simulink model "data_cap"  (R2013b)
settings: Solver=ode45  StartTime=0.0  StopTime=270000  RelTol=1e-3
undefined symbols (not defined in the file or in its folder): A, A2, B, D, EVAL, i, P, THIS_DATE, W, X, Z
libraries: xbsIndex_r4 x219, uram_lib x2
(part 1 of 2)
settings Model: Creator=ehngjun  LastModifiedBy=Administrator
settings GRTTargetCC: CodeReplacementLibrary=C89/C90 (ANSI)

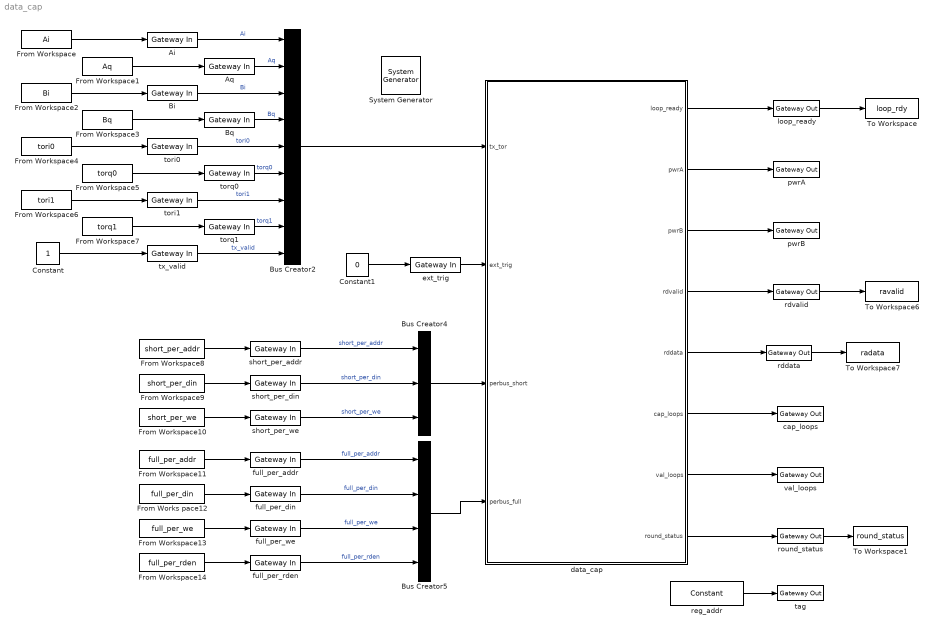
== system data_cap ==
  " System Generator" : xbsIndex_r4/ System Generator  Tag=genX  xilinxfamily=zynquplus  part=xczu15eg  speed=-1LV-i-EVAL  package=ffvb1156  synthesis_tool=Vivado  clock_wrapper=Clock Enables  directory=../../../netlist/datacap  proj_type=Vivado  Synth_file=Vivado Synthesis Defaults  Impl_file=Vivado Implementation Defaults  testbench=off  simulink_period=1  sysclk_period=3.2  dcm_input_clock_period=10  incr_netlist=off  trim_vbits=Everywhere in SubSystem  dbl_ovrd=According to Block Masks  core_generation=According to Block Masks  run_coregen=off  deprecated_control=off  eval_field=0  block_type=sysgen
  Ai : xbsIndex_r4/Gateway In  gui_display_data_type=Fixed-point  arith_type="Signed  (2's comp)"  n_bits=16  bin_pt=0  preci_type=Single  exp_width=8  frac_width=24  rows=1  columns=1  quantization="Round  (unbiased: +/- Inf)"  overflow=Saturate  period=1  UseAsADC=off  ADCChannel='1'  interface=None  automatic_assignment=on  address_offset=hex2dec('00')  intf_name=''  intf_description=''  default_value=0  timing_constraint=None  locs_specified=off  LOCs={}  io_standard={}  inherit_from_input=off  hdl_port=on  dbl_ovrd=off  block_type=gatewayin
  Aq : xbsIndex_r4/Gateway In  gui_display_data_type=Fixed-point  arith_type="Signed  (2's comp)"  n_bits=16  bin_pt=0  preci_type=Single  exp_width=8  frac_width=24  rows=1  columns=1  quantization="Round  (unbiased: +/- Inf)"  overflow=Saturate  period=1  UseAsADC=off  ADCChannel='1'  interface=None  automatic_assignment=on  address_offset=hex2dec('00')  intf_name=''  intf_description=''  default_value=0  timing_constraint=None  locs_specified=off  LOCs={}  io_standard={}  inherit_from_input=off  hdl_port=on  dbl_ovrd=off  block_type=gatewayin
  Bi : xbsIndex_r4/Gateway In  gui_display_data_type=Fixed-point  arith_type="Signed  (2's comp)"  n_bits=16  bin_pt=0  preci_type=Single  exp_width=8  frac_width=24  rows=1  columns=1  quantization="Round  (unbiased: +/- Inf)"  overflow=Saturate  period=1  UseAsADC=off  ADCChannel='1'  interface=None  automatic_assignment=on  address_offset=hex2dec('00')  intf_name=''  intf_description=''  default_value=0  timing_constraint=None  locs_specified=off  LOCs={}  io_standard={}  inherit_from_input=off  hdl_port=on  dbl_ovrd=off  block_type=gatewayin
  Bq : xbsIndex_r4/Gateway In  gui_display_data_type=Fixed-point  arith_type="Signed  (2's comp)"  n_bits=16  bin_pt=0  preci_type=Single  exp_width=8  frac_width=24  rows=1  columns=1  quantization="Round  (unbiased: +/- Inf)"  overflow=Saturate  period=1  UseAsADC=off  ADCChannel='1'  interface=None  automatic_assignment=on  address_offset=hex2dec('00')  intf_name=''  intf_description=''  default_value=0  timing_constraint=None  locs_specified=off  LOCs={}  io_standard={}  inherit_from_input=off  hdl_port=on  dbl_ovrd=off  block_type=gatewayin
  Bus Creator2 : BusCreator  Inputs=9
  Bus Creator4 : BusCreator  Inputs=3
  Bus Creator5 : BusCreator
  Constant : Constant
  Constant1 : Constant  Value=0
  From Works pace12 : FromWorkspace  VariableName=full_per_din  SampleTime=1  Interpolate=off  OutputAfterFinalValue=Setting to zero
  From Workspace : FromWorkspace  VariableName=Ai  SampleTime=1  Interpolate=off  OutputAfterFinalValue=Setting to zero
  From Workspace1 : FromWorkspace  VariableName=Aq  SampleTime=1  Interpolate=off  OutputAfterFinalValue=Setting to zero
  From Workspace10 : FromWorkspace  VariableName=short_per_we  SampleTime=1  Interpolate=off  OutputAfterFinalValue=Setting to zero
  From Workspace11 : FromWorkspace  VariableName=full_per_addr  SampleTime=1  Interpolate=off  OutputAfterFinalValue=Setting to zero
  From Workspace13 : FromWorkspace  VariableName=full_per_we  SampleTime=1  Interpolate=off  OutputAfterFinalValue=Setting to zero
  From Workspace14 : FromWorkspace  VariableName=full_per_rden  SampleTime=1  Interpolate=off  OutputAfterFinalValue=Setting to zero
  From Workspace2 : FromWorkspace  VariableName=Bi  SampleTime=1  Interpolate=off  OutputAfterFinalValue=Setting to zero
  From Workspace3 : FromWorkspace  VariableName=Bq  SampleTime=1  Interpolate=off  OutputAfterFinalValue=Setting to zero
  From Workspace4 : FromWorkspace  VariableName=tori0  SampleTime=1  Interpolate=off  OutputAfterFinalValue=Setting to zero
  From Workspace5 : FromWorkspace  VariableName=torq0  SampleTime=1  Interpolate=off  OutputAfterFinalValue=Setting to zero
  From Workspace6 : FromWorkspace  VariableName=tori1  SampleTime=1  Interpolate=off  OutputAfterFinalValue=Setting to zero
  From Workspace7 : FromWorkspace  VariableName=torq1  SampleTime=1  Interpolate=off  OutputAfterFinalValue=Setting to zero
  From Workspace8 : FromWorkspace  VariableName=short_per_addr  SampleTime=1  Interpolate=off  OutputAfterFinalValue=Setting to zero
  From Workspace9 : FromWorkspace  VariableName=short_per_din  SampleTime=1  Interpolate=off  OutputAfterFinalValue=Setting to zero
  To Workspace : ToWorkspace  VariableName=loop_rdy  SampleTime=-1
  To Workspace1 : ToWorkspace  VariableName=round_status  SampleTime=-1
  To Workspace6 : ToWorkspace  VariableName=ravalid  SampleTime=-1
  To Workspace7 : ToWorkspace  VariableName=radata  SampleTime=-1
  cap_loops : xbsIndex_r4/Gateway Out  inherit_from_input=off  hdl_port=on  rows=1  columns=1  UseAsDAC=off  DACChannel='1'  interface=None  automatic_assignment=on  address_offset=hex2dec('00')  intf_name=''  intf_description=''  timing_constraint=None  locs_specified=off  LOCs={}  io_standard={}  block_type=gatewayout
  data_cap : Subsystem
  ext_trig : xbsIndex_r4/Gateway In  gui_display_data_type=Boolean  arith_type=Boolean  n_bits=16  bin_pt=14  preci_type=Single  exp_width=8  frac_width=24  rows=1  columns=1  quantization="Round  (unbiased: +/- Inf)"  overflow=Saturate  period=1  UseAsADC=off  ADCChannel='1'  interface=None  automatic_assignment=on  address_offset=hex2dec('00')  intf_name=''  intf_description=''  default_value=0  timing_constraint=None  locs_specified=off  LOCs={}  io_standard={}  inherit_from_input=off  hdl_port=on  dbl_ovrd=off  block_type=gatewayin
  full_per_addr : xbsIndex_r4/Gateway In  gui_display_data_type=Fixed-point  arith_type=Unsigned  n_bits=20  bin_pt=0  preci_type=Single  exp_width=8  frac_width=24  rows=1  columns=1  quantization="Round  (unbiased: +/- Inf)"  overflow=Saturate  period=1  UseAsADC=off  ADCChannel='1'  interface=None  automatic_assignment=on  address_offset=hex2dec('00')  intf_name=''  intf_description=''  default_value=0  timing_constraint=None  locs_specified=off  LOCs={}  io_standard={}  inherit_from_input=off  hdl_port=on  dbl_ovrd=off  block_type=gatewayin
  full_per_din : xbsIndex_r4/Gateway In  gui_display_data_type=Fixed-point  arith_type=Unsigned  n_bits=32  bin_pt=0  preci_type=Single  exp_width=8  frac_width=24  rows=1  columns=1  quantization="Round  (unbiased: +/- Inf)"  overflow=Saturate  period=1  UseAsADC=off  ADCChannel='1'  interface=None  automatic_assignment=on  address_offset=hex2dec('00')  intf_name=''  intf_description=''  default_value=0  timing_constraint=None  locs_specified=off  LOCs={}  io_standard={}  inherit_from_input=off  hdl_port=on  dbl_ovrd=off  block_type=gatewayin
  full_per_rden : xbsIndex_r4/Gateway In  gui_display_data_type=Boolean  arith_type=Boolean  n_bits=16  bin_pt=0  preci_type=Single  exp_width=8  frac_width=24  rows=1  columns=1  quantization="Round  (unbiased: +/- Inf)"  overflow=Saturate  period=1  UseAsADC=off  ADCChannel='1'  interface=None  automatic_assignment=on  address_offset=hex2dec('00')  intf_name=''  intf_description=''  default_value=0  timing_constraint=None  locs_specified=off  LOCs={}  io_standard={}  inherit_from_input=off  hdl_port=on  dbl_ovrd=off  block_type=gatewayin
  full_per_we : xbsIndex_r4/Gateway In  gui_display_data_type=Boolean  arith_type=Boolean  n_bits=16  bin_pt=0  preci_type=Single  exp_width=8  frac_width=24  rows=1  columns=1  quantization="Round  (unbiased: +/- Inf)"  overflow=Saturate  period=1  UseAsADC=off  ADCChannel='1'  interface=None  automatic_assignment=on  address_offset=hex2dec('00')  intf_name=''  intf_description=''  default_value=0  timing_constraint=None  locs_specified=off  LOCs={}  io_standard={}  inherit_from_input=off  hdl_port=on  dbl_ovrd=off  block_type=gatewayin
  loop_ready : xbsIndex_r4/Gateway Out  inherit_from_input=off  hdl_port=on  rows=1  columns=1  UseAsDAC=off  DACChannel='1'  interface=None  automatic_assignment=on  address_offset=hex2dec('00')  intf_name=''  intf_description=''  timing_constraint=None  locs_specified=off  LOCs={}  io_standard={}  block_type=gatewayout
  pwrA : xbsIndex_r4/Gateway Out  inherit_from_input=off  hdl_port=on  rows=1  columns=1  UseAsDAC=off  DACChannel='1'  interface=None  automatic_assignment=on  address_offset=hex2dec('00')  intf_name=''  intf_description=''  timing_constraint=None  locs_specified=off  LOCs={}  io_standard={}  block_type=gatewayout
  pwrB : xbsIndex_r4/Gateway Out  inherit_from_input=off  hdl_port=on  rows=1  columns=1  UseAsDAC=off  DACChannel='1'  interface=None  automatic_assignment=on  address_offset=hex2dec('00')  intf_name=''  intf_description=''  timing_constraint=None  locs_specified=off  LOCs={}  io_standard={}  block_type=gatewayout
  rddata : xbsIndex_r4/Gateway Out  inherit_from_input=off  hdl_port=on  rows=1  columns=1  UseAsDAC=off  DACChannel='1'  interface=None  automatic_assignment=on  address_offset=hex2dec('00')  intf_name=''  intf_description=''  timing_constraint=None  locs_specified=off  LOCs={}  io_standard={}  block_type=gatewayout
  rdvalid : xbsIndex_r4/Gateway Out  inherit_from_input=off  hdl_port=on  rows=1  columns=1  UseAsDAC=off  DACChannel='1'  interface=None  automatic_assignment=on  address_offset=hex2dec('00')  intf_name=''  intf_description=''  timing_constraint=None  locs_specified=off  LOCs={}  io_standard={}  block_type=gatewayout
  reg_addr : xbsIndex_r4/Constant  const=THIS_DATE  gui_display_data_type=Fixed-point  arith_type=Unsigned  n_bits=32  bin_pt=0  preci_type=Single  exp_width=8  frac_width=24  explicit_period=off  period=1  equ=P=C  opselect=C  inp2=PCIN>>17  opr=+  inp1=P  carry=CIN  dbl_ovrd=off  block_type=constant
  round_status : xbsIndex_r4/Gateway Out  inherit_from_input=off  hdl_port=on  rows=1  columns=1  UseAsDAC=off  DACChannel='1'  interface=None  automatic_assignment=on  address_offset=hex2dec('00')  intf_name=''  intf_description=''  timing_constraint=None  locs_specified=off  LOCs={}  io_standard={}  block_type=gatewayout
  short_per_addr : xbsIndex_r4/Gateway In  gui_display_data_type=Fixed-point  arith_type=Unsigned  n_bits=12  bin_pt=0  preci_type=Single  exp_width=8  frac_width=24  rows=1  columns=1  quantization="Round  (unbiased: +/- Inf)"  overflow=Saturate  period=1  UseAsADC=off  ADCChannel='1'  interface=None  automatic_assignment=on  address_offset=hex2dec('00')  intf_name=''  intf_description=''  default_value=0  timing_constraint=None  locs_specified=off  LOCs={}  io_standard={}  inherit_from_input=off  hdl_port=on  dbl_ovrd=off  block_type=gatewayin
  short_per_din : xbsIndex_r4/Gateway In  gui_display_data_type=Fixed-point  arith_type=Unsigned  n_bits=32  bin_pt=0  preci_type=Single  exp_width=8  frac_width=24  rows=1  columns=1  quantization="Round  (unbiased: +/- Inf)"  overflow=Saturate  period=1  UseAsADC=off  ADCChannel='1'  interface=None  automatic_assignment=on  address_offset=hex2dec('00')  intf_name=''  intf_description=''  default_value=0  timing_constraint=None  locs_specified=off  LOCs={}  io_standard={}  inherit_from_input=off  hdl_port=on  dbl_ovrd=off  block_type=gatewayin
  short_per_we : xbsIndex_r4/Gateway In  gui_display_data_type=Boolean  arith_type=Boolean  n_bits=16  bin_pt=0  preci_type=Single  exp_width=8  frac_width=24  rows=1  columns=1  quantization="Round  (unbiased: +/- Inf)"  overflow=Saturate  period=1  UseAsADC=off  ADCChannel='1'  interface=None  automatic_assignment=on  address_offset=hex2dec('00')  intf_name=''  intf_description=''  default_value=0  timing_constraint=None  locs_specified=off  LOCs={}  io_standard={}  inherit_from_input=off  hdl_port=on  dbl_ovrd=off  block_type=gatewayin
  tag : xbsIndex_r4/Gateway Out  inherit_from_input=off  hdl_port=on  rows=1  columns=1  UseAsDAC=off  DACChannel='1'  interface=None  automatic_assignment=on  address_offset=hex2dec('00')  intf_name=''  intf_description=''  timing_constraint=None  locs_specified=off  LOCs={}  io_standard={}  block_type=gatewayout
  tori0 : xbsIndex_r4/Gateway In  gui_display_data_type=Fixed-point  arith_type="Signed  (2's comp)"  n_bits=16  bin_pt=0  preci_type=Single  exp_width=8  frac_width=24  rows=1  columns=1  quantization="Round  (unbiased: +/- Inf)"  overflow=Saturate  period=1  UseAsADC=off  ADCChannel='1'  interface=None  automatic_assignment=on  address_offset=hex2dec('00')  intf_name=''  intf_description=''  default_value=0  timing_constraint=None  locs_specified=off  LOCs={}  io_standard={}  inherit_from_input=off  hdl_port=on  dbl_ovrd=off  block_type=gatewayin
  tori1 : xbsIndex_r4/Gateway In  gui_display_data_type=Fixed-point  arith_type="Signed  (2's comp)"  n_bits=16  bin_pt=0  preci_type=Single  exp_width=8  frac_width=24  rows=1  columns=1  quantization="Round  (unbiased: +/- Inf)"  overflow=Saturate  period=1  UseAsADC=off  ADCChannel='1'  interface=None  automatic_assignment=on  address_offset=hex2dec('00')  intf_name=''  intf_description=''  default_value=0  timing_constraint=None  locs_specified=off  LOCs={}  io_standard={}  inherit_from_input=off  hdl_port=on  dbl_ovrd=off  block_type=gatewayin
  torq0 : xbsIndex_r4/Gateway In  gui_display_data_type=Fixed-point  arith_type="Signed  (2's comp)"  n_bits=16  bin_pt=0  preci_type=Single  exp_width=8  frac_width=24  rows=1  columns=1  quantization="Round  (unbiased: +/- Inf)"  overflow=Saturate  period=1  UseAsADC=off  ADCChannel='1'  interface=None  automatic_assignment=on  address_offset=hex2dec('00')  intf_name=''  intf_description=''  default_value=0  timing_constraint=None  locs_specified=off  LOCs={}  io_standard={}  inherit_from_input=off  hdl_port=on  dbl_ovrd=off  block_type=gatewayin
  torq1 : xbsIndex_r4/Gateway In  gui_display_data_type=Fixed-point  arith_type="Signed  (2's comp)"  n_bits=16  bin_pt=0  preci_type=Single  exp_width=8  frac_width=24  rows=1  columns=1  quantization="Round  (unbiased: +/- Inf)"  overflow=Saturate  period=1  UseAsADC=off  ADCChannel='1'  interface=None  automatic_assignment=on  address_offset=hex2dec('00')  intf_name=''  intf_description=''  default_value=0  timing_constraint=None  locs_specified=off  LOCs={}  io_standard={}  inherit_from_input=off  hdl_port=on  dbl_ovrd=off  block_type=gatewayin
  tx_valid : xbsIndex_r4/Gateway In  gui_display_data_type=Boolean  arith_type=Boolean  n_bits=16  bin_pt=14  preci_type=Single  exp_width=8  frac_width=24  rows=1  columns=1  quantization="Round  (unbiased: +/- Inf)"  overflow=Saturate  period=1  UseAsADC=off  ADCChannel='1'  interface=None  automatic_assignment=on  address_offset=hex2dec('00')  intf_name=''  intf_description=''  default_value=0  timing_constraint=None  locs_specified=off  LOCs={}  io_standard={}  inherit_from_input=off  hdl_port=on  dbl_ovrd=off  block_type=gatewayin
  val_loops : xbsIndex_r4/Gateway Out  inherit_from_input=off  hdl_port=on  rows=1  columns=1  UseAsDAC=off  DACChannel='1'  interface=None  automatic_assignment=on  address_offset=hex2dec('00')  intf_name=''  intf_description=''  timing_constraint=None  locs_specified=off  LOCs={}  io_standard={}  block_type=gatewayout
  wires:
  Ai/1 -> Bus Creator2/1  "Ai"
  Bi/1 -> Bus Creator2/3  "Bi"
  tori0/1 -> Bus Creator2/5  "tori0"
  tori1/1 -> Bus Creator2/7  "tori1"
  Aq/1 -> Bus Creator2/2  "Aq"
  Bq/1 -> Bus Creator2/4  "Bq"
  torq0/1 -> Bus Creator2/6  "torq0"
  torq1/1 -> Bus Creator2/8  "torq1"
  tx_valid/1 -> Bus Creator2/9  "tx_valid"
  Bus Creator2/1 -> data_cap/1(tx_tor)
  ext_trig/1 -> data_cap/2(ext_trig)
  data_cap/8(round_status) -> round_status/1
  data_cap/6(cap_loops) -> cap_loops/1
  data_cap/7(val_loops) -> val_loops/1
  data_cap/2(pwrA) -> pwrA/1
  From Workspace/1 -> Ai/1
  From Workspace1/1 -> Aq/1
  From Workspace2/1 -> Bi/1
  From Workspace3/1 -> Bq/1
  From Workspace4/1 -> tori0/1
  From Workspace5/1 -> torq0/1
  From Workspace6/1 -> tori1/1
  From Workspace7/1 -> torq1/1
  Constant1/1 -> ext_trig/1
  loop_ready/1 -> To Workspace/1
  round_status/1 -> To Workspace1/1
  Constant/1 -> tx_valid/1
  data_cap/3(pwrB) -> pwrB/1
  short_per_addr/1 -> Bus Creator4/1  "short_per_addr"
  short_per_din/1 -> Bus Creator4/2  "short_per_din"
  short_per_we/1 -> Bus Creator4/3  "short_per_we"
  Bus Creator4/1 -> data_cap/3(perbus_short)
  full_per_addr/1 -> Bus Creator5/1  "full_per_addr"
  full_per_din/1 -> Bus Creator5/2  "full_per_din"
  full_per_we/1 -> Bus Creator5/3  "full_per_we"
  Bus Creator5/1 -> data_cap/4(perbus_full)
  data_cap/4(rdvalid) -> rdvalid/1
  rdvalid/1 -> To Workspace6/1
  From Workspace8/1 -> short_per_addr/1
  From Workspace9/1 -> short_per_din/1
  From Workspace10/1 -> short_per_we/1
  From Workspace11/1 -> full_per_addr/1
  From Works pace12/1 -> full_per_din/1
  From Workspace13/1 -> full_per_we/1
  data_cap/1(loop_ready) -> loop_ready/1
  data_cap/5(rddata) -> rddata/1
  rddata/1 -> To Workspace7/1
  From Workspace14/1 -> full_per_rden/1
  full_per_rden/1 -> Bus Creator5/4  "full_per_rden"
  reg_addr/1 -> tag/1

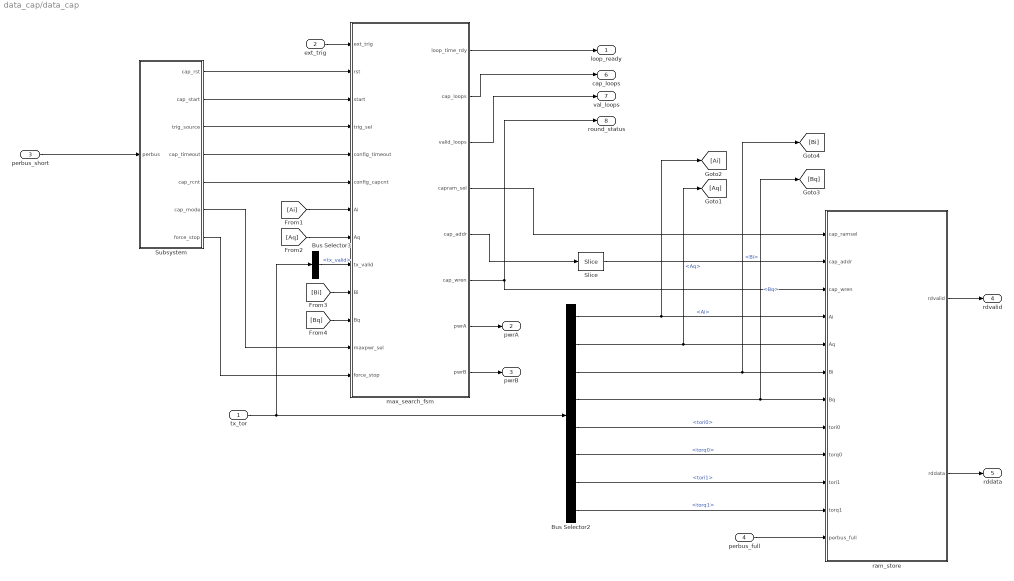
== system data_cap/data_cap ==
  tx_tor : Inport
  ext_trig : Inport  Port=2
  perbus_short : Inport  Port=3
  perbus_full : Inport  Port=4
  Bus Selector2 : BusSelector  OutputSignals=Ai,Aq,Bi,Bq,tori0,torq0,tori1,torq1
  Bus Selector3 : BusSelector  OutputSignals=tx_valid
  Slice : xbsIndex_r4/Slice  nbits=15  boolean_output=off  mode=Lower Bit Location + Width  bit1=0  base1=MSB of Input  bit0=0  base0=LSB of Input  dbl_ovrd=off  block_type=slice
  Subsystem : Subsystem
  max_search_fsm : Subsystem
  ram_store : Subsystem
  loop_ready : Outport
  pwrA : Outport  Port=2
  pwrB : Outport  Port=3
  rdvalid : Outport  Port=4
  rddata : Outport  Port=5
  cap_loops : Outport  Port=6
  val_loops : Outport  Port=7
  round_status : Outport  Port=8
  wires:
  Bus Selector3/1 -> max_search_fsm/9(tx_valid)  "<tx_valid>"
  [Aq] -> max_search_fsm/8(Aq)
  [Ai] -> max_search_fsm/7(Ai)
  Bus Selector2/5 -> ram_store/8(tori0)  "<tori0>"
  Bus Selector2/4 -> [Bq], ram_store/7(Bq)  "<Bq>"
  Bus Selector2/3 -> [Bi], ram_store/6(Bi)  "<Bi>"
  Bus Selector2/2 -> [Aq], ram_store/5(Aq)  "<Aq>"
  Bus Selector2/1 -> [Ai], ram_store/4(Ai)  "<Ai>"
  tx_tor/1 -> Bus Selector2/1, Bus Selector3/1
  Slice/1 -> ram_store/2(cap_addr)
  max_search_fsm/6(cap_wren) -> round_status/1, ram_store/3(cap_wren)
  max_search_fsm/5(cap_addr) -> Slice/1
  max_search_fsm/4(capram_sel) -> ram_store/1(cap_ramsel)
  max_search_fsm/3(valid_loops) -> val_loops/1
  max_search_fsm/2(cap_loops) -> cap_loops/1
  max_search_fsm/1(loop_time_rdy) -> loop_ready/1
  Subsystem/5(cap_rcnt) -> max_search_fsm/6(config_capcnt)
  Subsystem/4(cap_timeout) -> max_search_fsm/5(config_timeout)
  ext_trig/1 -> max_search_fsm/1(ext_trig)
  Subsystem/3(trig_source) -> max_search_fsm/4(trig_sel)
  Subsystem/2(cap_start) -> max_search_fsm/3(start)
  Bus Selector2/6 -> ram_store/9(torq0)  "<torq0>"
  Bus Selector2/7 -> ram_store/10(tori1)  "<tori1>"
  Bus Selector2/8 -> ram_store/11(torq1)  "<torq1>"
  [Bi] -> max_search_fsm/10(Bi)
  [Bq] -> max_search_fsm/11(Bq)
  Subsystem/6(cap_mode) -> max_search_fsm/12(maxpwr_sel)
  Subsystem/7(force_stop) -> max_search_fsm/13(force_stop)
  max_search_fsm/7(pwrA) -> pwrA/1
  max_search_fsm/8(pwrB) -> pwrB/1
  perbus_short/1 -> Subsystem/1(perbus)
  perbus_full/1 -> ram_store/12(perbus_full)
  ram_store/1(rdvalid) -> rdvalid/1
  ram_store/2(rddata) -> rddata/1
  Subsystem/1(cap_rst) -> max_search_fsm/2(rst)

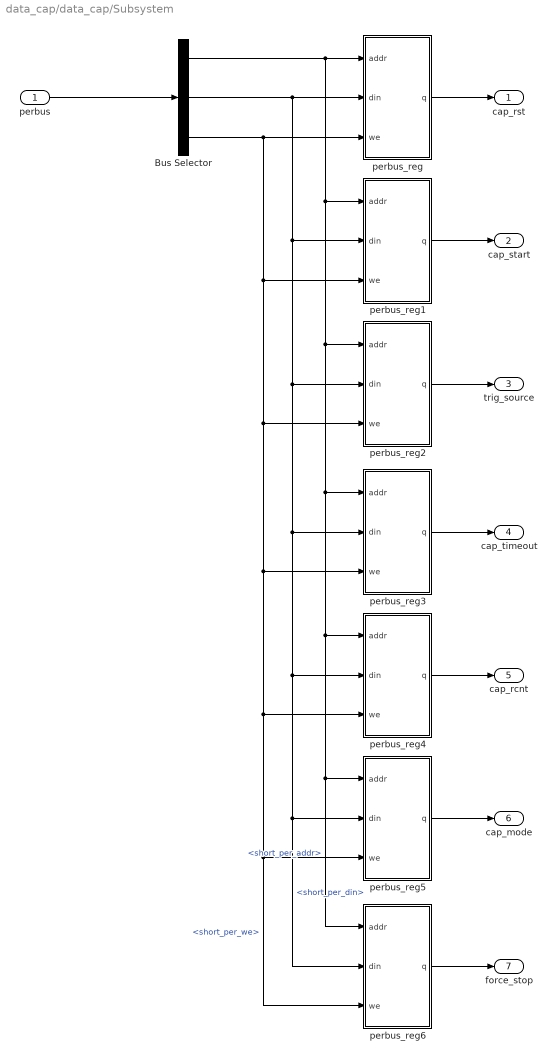
== system data_cap/data_cap/Subsystem ==
  perbus : Inport
  Bus Selector : BusSelector  OutputSignals=short_per_addr,short_per_din,short_per_we
  perbus_reg : Subsystem  mask{reg_addr=hex2dec('150')}
      mask prompts: reg_addr "cap_rst"
  perbus_reg1 : Subsystem  mask{reg_addr=hex2dec('150')}
      mask prompts: reg_addr "cap_start"
  perbus_reg2 : Subsystem  mask{reg_addr=hex2dec('150')}
      mask prompts: reg_addr "trig_source"
  perbus_reg3 : Subsystem  mask{reg_addr=hex2dec('152')}
      mask prompts: reg_addr "cap_timeout"
  perbus_reg4 : Subsystem  mask{reg_addr=hex2dec('151')}
      mask prompts: reg_addr "cap_rcnt"
  perbus_reg5 : Subsystem  mask{reg_addr=hex2dec('150')}
      mask prompts: reg_addr "cap_mode"
  perbus_reg6 : Subsystem  mask{reg_addr=hex2dec('150')}
      mask prompts: reg_addr "force_stop"
  cap_rst : Outport
  cap_start : Outport  Port=2
  trig_source : Outport  Port=3
  cap_timeout : Outport  Port=4
  cap_rcnt : Outport  Port=5
  cap_mode : Outport  Port=6
  force_stop : Outport  Port=7
  wires:
  perbus_reg/1(q) -> cap_rst/1
  Bus Selector/3 -> perbus_reg3/3(we), perbus_reg6/3(we), perbus_reg5/3(we), perbus_reg4/3(we), perbus_reg2/3(we), perbus_reg1/3(we), perbus_reg/3(we)  "<short_per_we>"
  Bus Selector/2 -> perbus_reg6/2(din), perbus_reg5/2(din), perbus_reg4/2(din), perbus_reg3/2(din), perbus_reg2/2(din), perbus_reg1/2(din), perbus_reg/2(din)  "<short_per_din>"
  Bus Selector/1 -> perbus_reg6/1(addr), perbus_reg5/1(addr), perbus_reg4/1(addr), perbus_reg3/1(addr), perbus_reg2/1(addr), perbus_reg1/1(addr), perbus_reg/1(addr)  "<short_per_addr>"
  perbus/1 -> Bus Selector/1
  perbus_reg6/1(q) -> force_stop/1
  perbus_reg5/1(q) -> cap_mode/1
  perbus_reg4/1(q) -> cap_rcnt/1
  perbus_reg1/1(q) -> cap_start/1
  perbus_reg2/1(q) -> trig_source/1
  perbus_reg3/1(q) -> cap_timeout/1

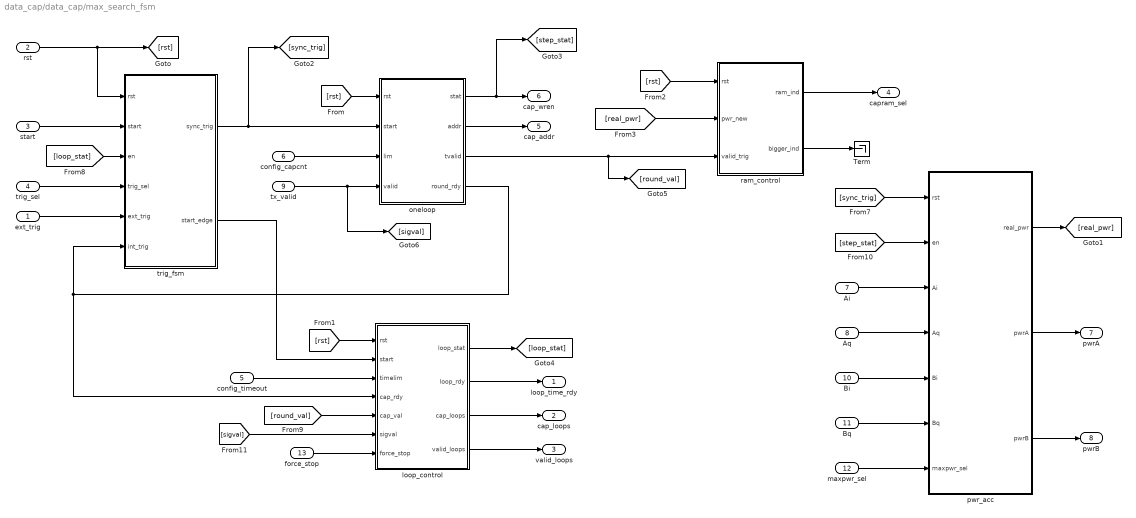
== system data_cap/data_cap/max_search_fsm ==
  ext_trig : Inport
  rst : Inport  Port=2
  start : Inport  Port=3
  trig_sel : Inport  Port=4
  config_timeout : Inport  Port=5
  config_capcnt : Inport  Port=6
  Ai : Inport  Port=7
  Aq : Inport  Port=8
  tx_valid : Inport  Port=9
  Bi : Inport  Port=10
  Bq : Inport  Port=11
  maxpwr_sel : Inport  Port=12
  force_stop : Inport  Port=13
  Term : Terminator
  loop_control : Subsystem
  oneloop : Subsystem
  pwr_acc : Subsystem
  ram_control : Subsystem
  trig_fsm : Subsystem
  loop_time_rdy : Outport
  cap_loops : Outport  Port=2
  valid_loops : Outport  Port=3
  capram_sel : Outport  Port=4
  cap_addr : Outport  Port=5
  cap_wren : Outport  Port=6
  pwrA : Outport  Port=7
  pwrB : Outport  Port=8
  wires:
  [step_stat] -> pwr_acc/2(en)
  tx_valid/1 -> [sigval], oneloop/4(valid)
  loop_control/4(valid_loops) -> valid_loops/1
  loop_control/3(cap_loops) -> cap_loops/1
  loop_control/2(loop_rdy) -> loop_time_rdy/1
  oneloop/1(stat) -> [step_stat], cap_wren/1
  oneloop/2(addr) -> cap_addr/1
  ram_control/2(bigger_ind) -> Term/1
  [round_val] -> loop_control/5(cap_val)
  [loop_stat] -> trig_fsm/3(en)
  loop_control/1(loop_stat) -> [loop_stat]
  Aq/1 -> pwr_acc/4(Aq)
  Ai/1 -> pwr_acc/3(Ai)
  [real_pwr] -> ram_control/2(pwr_new)
  pwr_acc/1(real_pwr) -> [real_pwr]
  oneloop/3(tvalid) -> ram_control/3(valid_trig), [round_val]
  [rst] -> ram_control/1(rst)
  config_timeout/1 -> loop_control/3(timelim)
  [rst] -> loop_control/1(rst)
  [rst] -> oneloop/1(rst)
  oneloop/4(round_rdy) -> loop_control/4(cap_rdy), trig_fsm/6(int_trig)
  config_capcnt/1 -> oneloop/3(lim)
  trig_fsm/1(sync_trig) -> oneloop/2(start), [sync_trig]
  ext_trig/1 -> trig_fsm/5(ext_trig)
  trig_sel/1 -> trig_fsm/4(trig_sel)
  start/1 -> trig_fsm/2(start)
  rst/1 -> trig_fsm/1(rst), [rst]
  [sigval] -> loop_control/6(sigval)
  Bi/1 -> pwr_acc/5(Bi)
  Bq/1 -> pwr_acc/6(Bq)
  maxpwr_sel/1 -> pwr_acc/7(maxpwr_sel)
  force_stop/1 -> loop_control/7(force_stop)
  pwr_acc/2(pwrA) -> pwrA/1
  pwr_acc/3(pwrB) -> pwrB/1
  trig_fsm/2(start_edge) -> loop_control/2(start)
  ram_control/1(ram_ind) -> capram_sel/1
  [sync_trig] -> pwr_acc/1(rst)

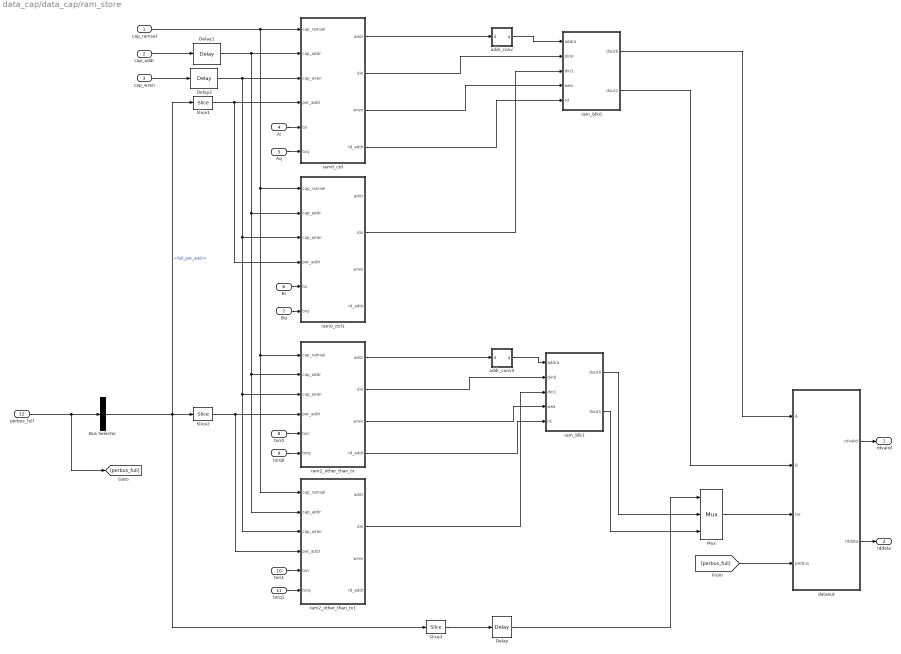
== system data_cap/data_cap/ram_store ==
  cap_ramsel : Inport
  cap_addr : Inport  Port=2
  cap_wren : Inport  Port=3
  Ai : Inport  Port=4
  Aq : Inport  Port=5
  Bi : Inport  Port=6
  Bq : Inport  Port=7
  tori0 : Inport  Port=8
  torq0 : Inport  Port=9
  tori1 : Inport  Port=10
  torq1 : Inport  Port=11
  perbus_full : Inport  Port=12
  Bus Selector : BusSelector  OutputSignals=full_per_addr
  Delay : xbsIndex_r4/Delay  rst=off  infoeditControl=Selection of Reset will increase slice count due to use of real FFs and instead of SRLs  en=off  latency=12  reg_retiming=off  dbl_ovrd=off  block_type=delay
  Delay1 : xbsIndex_r4/Delay  rst=off  infoeditControl=Selection of Reset will increase slice count due to use of real FFs and instead of SRLs  en=off  latency=1  reg_retiming=off  dbl_ovrd=off  block_type=delay
  Delay2 : xbsIndex_r4/Delay  rst=off  infoeditControl=Selection of Reset will increase slice count due to use of real FFs and instead of SRLs  en=off  latency=1  reg_retiming=off  dbl_ovrd=off  block_type=delay
  Mux : xbsIndex_r4/Mux  inputs=2  en=off  latency=0  precision=Full  arith_type=Unsigned  n_bits=16  bin_pt=14  quantization=Truncate  overflow=Wrap  dbl_ovrd=off  block_type=mux
  Slice1 : xbsIndex_r4/Slice  nbits=14  boolean_output=off  mode=Lower Bit Location + Width  bit1=0  base1=MSB of Input  bit0=0  base0=LSB of Input  dbl_ovrd=off  block_type=slice
  Slice2 : xbsIndex_r4/Slice  nbits=14  boolean_output=off  mode=Lower Bit Location + Width  bit1=0  base1=MSB of Input  bit0=1  base0=LSB of Input  dbl_ovrd=off  block_type=slice
  Slice3 : xbsIndex_r4/Slice  nbits=1  boolean_output=off  mode=Lower Bit Location + Width  bit1=0  base1=MSB of Input  bit0=0  base0=LSB of Input  dbl_ovrd=off  block_type=slice
  addr_conv : Subsystem  mask{cap_addr_width=14}
  addr_conv5 : Subsystem  mask{cap_addr_width=14}
  dataout : Subsystem
  ram0_ctrl : Subsystem
  ram0_ctrl1 : Subsystem
  ram2_other_than_tx : Subsystem
  ram2_other_than_tx1 : Subsystem
  ram_blk0 : Subsystem
  ram_blk1 : Subsystem
  rdvalid : Outport
  rddata : Outport  Port=2
  wires:
  Slice1/1 -> ram0_ctrl1/4(per_addr), ram0_ctrl/4(per_addr)
  ram2_other_than_tx/3(wren) -> ram_blk1/4(wea)
  ram2_other_than_tx/1(addr) -> addr_conv5/1(d)
  tori0/1 -> ram2_other_than_tx/5(tori)
  cap_ramsel/1 -> ram2_other_than_tx1/1(cap_ramsel), ram2_other_than_tx/1(cap_ramsel), ram0_ctrl1/1(cap_ramsel), ram0_ctrl/1(cap_ramsel)
  ram0_ctrl/3(wren) -> ram_blk0/4(wea)
  ram0_ctrl/2(din) -> ram_blk0/2(din0)
  ram0_ctrl/1(addr) -> addr_conv/1(d)
  Bq/1 -> ram0_ctrl1/6(txq)
  Bi/1 -> ram0_ctrl1/5(txi)
  Aq/1 -> ram0_ctrl/6(txq)
  cap_wren/1 -> Delay2/1
  addr_conv/1(q) -> ram_blk0/1(addra)
  ram2_other_than_tx/2(din) -> ram_blk1/2(din0)
  addr_conv5/1(q) -> ram_blk1/1(addra)
  ram2_other_than_tx/4(rd_addr) -> ram_blk1/5(rd)
  torq0/1 -> ram2_other_than_tx/6(torq)
  tori1/1 -> ram2_other_than_tx1/5(tori)
  torq1/1 -> ram2_other_than_tx1/6(torq)
  ram2_other_than_tx1/2(din) -> ram_blk1/3(din1)
  ram0_ctrl/4(rd_addr) -> ram_blk0/5(rd)
  Slice2/1 -> ram2_other_than_tx1/4(per_addr), ram2_other_than_tx/4(per_addr)
  dataout/2(rddata) -> rddata/1
  [perbus_full] -> dataout/4(perbus)
  ram_blk0/2(dout1) -> dataout/2(B)
  dataout/1(rdvalid) -> rdvalid/1
  perbus_full/1 -> [perbus_full], Bus Selector/1
  Bus Selector/1 -> Slice1/1, Slice3/1, Slice2/1  "<full_per_addr>"
  Slice3/1 -> Delay/1
  ram_blk1/1(dout0) -> Mux/2
  Mux/1 -> dataout/3(tor)
  Delay/1 -> Mux/1
  ram_blk0/1(dout0) -> dataout/1(A)
  Ai/1 -> ram0_ctrl/5(txi)
  Delay1/1 -> ram0_ctrl1/2(cap_addr), ram2_other_than_tx1/2(cap_addr), ram2_other_than_tx/2(cap_addr), ram0_ctrl/2(cap_addr)
  Delay2/1 -> ram0_ctrl1/3(cap_wren), ram2_other_than_tx1/3(cap_wren), ram2_other_than_tx/3(cap_wren), ram0_ctrl/3(cap_wren)
  ram_blk1/2(dout1) -> Mux/3
  cap_addr/1 -> Delay1/1
  ram0_ctrl1/2(din) -> ram_blk0/3(din1)

== system data_cap/data_cap/Subsystem/perbus_reg ==
  addr : Inport
  din : Inport  Port=2
  we : Inport  Port=3
  Logical : xbsIndex_r4/Logical  logical_function=AND  inputs=2  en=off  latency=0  precision=Full  arith_type=Unsigned  n_bits=16  bin_pt=0  align_bp=on  dbl_ovrd=off  block_type=logical
  Register : xbsIndex_r4/Register  init=0  rst=off  en=on  dbl_ovrd=off  block_type=register
  Relational : xbsIndex_r4/Relational  mode=a=b  op_type=Bool  en=off  latency=0  dbl_ovrd=off  block_type=relational
  bit[1] : xbsIndex_r4/Slice  nbits=1  boolean_output=on  mode=Lower Bit Location + Width  bit1=0  base1=MSB of Input  bit0=1  base0=LSB of Input  dbl_ovrd=off  block_type=slice
  reg_addr : xbsIndex_r4/Constant  const=reg_addr  gui_display_data_type=Fixed-point  arith_type=Unsigned  n_bits=12  bin_pt=0  preci_type=Single  exp_width=8  frac_width=24  explicit_period=off  period=1  equ=P=C  opselect=C  inp2=PCIN>>17  opr=+  inp1=P  carry=CIN  dbl_ovrd=off  block_type=constant
  q : Outport
  wires:
  reg_addr/1 -> Relational/2
  addr/1 -> Relational/1
  Relational/1 -> Logical/2
  we/1 -> Logical/1
  Logical/1 -> Register/2
  din/1 -> bit[1]/1
  Register/1 -> q/1
  bit[1]/1 -> Register/1

== system data_cap/data_cap/Subsystem/perbus_reg1 ==
  addr : Inport
  din : Inport  Port=2
  we : Inport  Port=3
  Logical : xbsIndex_r4/Logical  logical_function=AND  inputs=2  en=off  latency=0  precision=Full  arith_type=Unsigned  n_bits=16  bin_pt=0  align_bp=on  dbl_ovrd=off  block_type=logical
  Register : xbsIndex_r4/Register  init=0  rst=off  en=on  dbl_ovrd=off  block_type=register
  Relational : xbsIndex_r4/Relational  mode=a=b  op_type=Bool  en=off  latency=0  dbl_ovrd=off  block_type=relational
  bit[2] : xbsIndex_r4/Slice  nbits=1  boolean_output=on  mode=Lower Bit Location + Width  bit1=0  base1=MSB of Input  bit0=2  base0=LSB of Input  dbl_ovrd=off  block_type=slice
  reg_addr : xbsIndex_r4/Constant  const=reg_addr  gui_display_data_type=Fixed-point  arith_type=Unsigned  n_bits=12  bin_pt=0  preci_type=Single  exp_width=8  frac_width=24  explicit_period=off  period=1  equ=P=C  opselect=C  inp2=PCIN>>17  opr=+  inp1=P  carry=CIN  dbl_ovrd=off  block_type=constant
  q : Outport
  wires:
  Register/1 -> q/1
  din/1 -> bit[2]/1
  Logical/1 -> Register/2
  we/1 -> Logical/1
  Relational/1 -> Logical/2
  addr/1 -> Relational/1
  reg_addr/1 -> Relational/2
  bit[2]/1 -> Register/1

== system data_cap/data_cap/Subsystem/perbus_reg2 ==
  addr : Inport
  din : Inport  Port=2
  we : Inport  Port=3
  Logical : xbsIndex_r4/Logical  logical_function=AND  inputs=2  en=off  latency=0  precision=Full  arith_type=Unsigned  n_bits=16  bin_pt=0  align_bp=on  dbl_ovrd=off  block_type=logical
  Register : xbsIndex_r4/Register  init=0  rst=off  en=on  dbl_ovrd=off  block_type=register
  Relational : xbsIndex_r4/Relational  mode=a=b  op_type=Bool  en=off  latency=0  dbl_ovrd=off  block_type=relational
  bit[0] : xbsIndex_r4/Slice  nbits=1  boolean_output=on  mode=Lower Bit Location + Width  bit1=0  base1=MSB of Input  bit0=0  base0=LSB of Input  dbl_ovrd=off  block_type=slice
  reg_addr : xbsIndex_r4/Constant  const=reg_addr  gui_display_data_type=Fixed-point  arith_type=Unsigned  n_bits=12  bin_pt=0  preci_type=Single  exp_width=8  frac_width=24  explicit_period=off  period=1  equ=P=C  opselect=C  inp2=PCIN>>17  opr=+  inp1=P  carry=CIN  dbl_ovrd=off  block_type=constant
  q : Outport
  wires:
  reg_addr/1 -> Relational/2
  addr/1 -> Relational/1
  Relational/1 -> Logical/2
  we/1 -> Logical/1
  Logical/1 -> Register/2
  din/1 -> bit[0]/1
  Register/1 -> q/1
  bit[0]/1 -> Register/1

== system data_cap/data_cap/Subsystem/perbus_reg3 ==
  addr : Inport
  din : Inport  Port=2
  we : Inport  Port=3
  Logical : xbsIndex_r4/Logical  logical_function=AND  inputs=2  en=off  latency=0  precision=Full  arith_type=Unsigned  n_bits=16  bin_pt=0  align_bp=on  dbl_ovrd=off  block_type=logical
  Register : xbsIndex_r4/Register  init=0  rst=off  en=on  dbl_ovrd=off  block_type=register
  Relational : xbsIndex_r4/Relational  mode=a=b  op_type=Bool  en=off  latency=0  dbl_ovrd=off  block_type=relational
  reg_addr : xbsIndex_r4/Constant  const=reg_addr  gui_display_data_type=Fixed-point  arith_type=Unsigned  n_bits=12  bin_pt=0  preci_type=Single  exp_width=8  frac_width=24  explicit_period=off  period=1  equ=P=C  opselect=C  inp2=PCIN>>17  opr=+  inp1=P  carry=CIN  dbl_ovrd=off  block_type=constant
  q : Outport
  wires:
  Register/1 -> q/1
  din/1 -> Register/1
  Logical/1 -> Register/2
  we/1 -> Logical/1
  Relational/1 -> Logical/2
  addr/1 -> Relational/1
  reg_addr/1 -> Relational/2

== system data_cap/data_cap/Subsystem/perbus_reg4 ==
  addr : Inport
  din : Inport  Port=2
  we : Inport  Port=3
  Logical : xbsIndex_r4/Logical  logical_function=AND  inputs=2  en=off  latency=0  precision=Full  arith_type=Unsigned  n_bits=16  bin_pt=0  align_bp=on  dbl_ovrd=off  block_type=logical
  Register : xbsIndex_r4/Register  init=0  rst=off  en=on  dbl_ovrd=off  block_type=register
  Relational : xbsIndex_r4/Relational  mode=a=b  op_type=Bool  en=off  latency=0  dbl_ovrd=off  block_type=relational
  reg_addr : xbsIndex_r4/Constant  const=reg_addr  gui_display_data_type=Fixed-point  arith_type=Unsigned  n_bits=12  bin_pt=0  preci_type=Single  exp_width=8  frac_width=24  explicit_period=off  period=1  equ=P=C  opselect=C  inp2=PCIN>>17  opr=+  inp1=P  carry=CIN  dbl_ovrd=off  block_type=constant
  q : Outport
  wires:
  reg_addr/1 -> Relational/2
  addr/1 -> Relational/1
  Relational/1 -> Logical/2
  we/1 -> Logical/1
  Logical/1 -> Register/2
  din/1 -> Register/1
  Register/1 -> q/1

== system data_cap/data_cap/Subsystem/perbus_reg5 ==
  addr : Inport
  din : Inport  Port=2
  we : Inport  Port=3
  Logical : xbsIndex_r4/Logical  logical_function=AND  inputs=2  en=off  latency=0  precision=Full  arith_type=Unsigned  n_bits=16  bin_pt=0  align_bp=on  dbl_ovrd=off  block_type=logical
  Register : xbsIndex_r4/Register  init=0  rst=off  en=on  dbl_ovrd=off  block_type=register
  Relational : xbsIndex_r4/Relational  mode=a=b  op_type=Bool  en=off  latency=0  dbl_ovrd=off  block_type=relational
  bit[5-4] : xbsIndex_r4/Slice  nbits=2  boolean_output=off  mode=Lower Bit Location + Width  bit1=0  base1=MSB of Input  bit0=4  base0=LSB of Input  dbl_ovrd=off  block_type=slice
  reg_addr : xbsIndex_r4/Constant  const=reg_addr  gui_display_data_type=Fixed-point  arith_type=Unsigned  n_bits=12  bin_pt=0  preci_type=Single  exp_width=8  frac_width=24  explicit_period=off  period=1  equ=P=C  opselect=C  inp2=PCIN>>17  opr=+  inp1=P  carry=CIN  dbl_ovrd=off  block_type=constant
  q : Outport
  wires:
  Register/1 -> q/1
  din/1 -> bit[5-4]/1
  Logical/1 -> Register/2
  we/1 -> Logical/1
  Relational/1 -> Logical/2
  addr/1 -> Relational/1
  reg_addr/1 -> Relational/2
  bit[5-4]/1 -> Register/1

== system data_cap/data_cap/Subsystem/perbus_reg6 ==
  addr : Inport
  din : Inport  Port=2
  we : Inport  Port=3
  Logical : xbsIndex_r4/Logical  logical_function=AND  inputs=2  en=off  latency=0  precision=Full  arith_type=Unsigned  n_bits=16  bin_pt=0  align_bp=on  dbl_ovrd=off  block_type=logical
  Register : xbsIndex_r4/Register  init=0  rst=off  en=on  dbl_ovrd=off  block_type=register
  Relational : xbsIndex_r4/Relational  mode=a=b  op_type=Bool  en=off  latency=0  dbl_ovrd=off  block_type=relational
  bit[2] : xbsIndex_r4/Slice  nbits=1  boolean_output=on  mode=Lower Bit Location + Width  bit1=0  base1=MSB of Input  bit0=3  base0=LSB of Input  dbl_ovrd=off  block_type=slice
  reg_addr : xbsIndex_r4/Constant  const=reg_addr  gui_display_data_type=Fixed-point  arith_type=Unsigned  n_bits=12  bin_pt=0  preci_type=Single  exp_width=8  frac_width=24  explicit_period=off  period=1  equ=P=C  opselect=C  inp2=PCIN>>17  opr=+  inp1=P  carry=CIN  dbl_ovrd=off  block_type=constant
  q : Outport
  wires:
  reg_addr/1 -> Relational/2
  addr/1 -> Relational/1
  Relational/1 -> Logical/2
  we/1 -> Logical/1
  Logical/1 -> Register/2
  din/1 -> bit[2]/1
  Register/1 -> q/1
  bit[2]/1 -> Register/1

== system data_cap/data_cap/max_search_fsm/loop_control ==
  rst : Inport
  start : Inport  Port=2
  timelim : Inport  Port=3
  cap_rdy : Inport  Port=4
  cap_val : Inport  Port=5
  sigval : Inport  Port=6
  force_stop : Inport  Port=7
  cap_loop : xbsIndex_r4/Counter  cnt_type=Free Running  cnt_to=Inf  operation=Up  start_count=0  cnt_by_val=1  arith_type=Unsigned  n_bits=16  bin_pt=0  load_pin=off  rst=on  en=on  explicit_period=on  period=1  use_behavioral_HDL=off  implementation=Fabric  dbl_ovrd=off  block_type=counter
  time_counters : Subsystem
  valid_loop : xbsIndex_r4/Counter  cnt_type=Free Running  cnt_to=Inf  operation=Up  start_count=0  cnt_by_val=1  arith_type=Unsigned  n_bits=16  bin_pt=0  load_pin=off  rst=on  en=on  explicit_period=on  period=1  use_behavioral_HDL=off  implementation=Fabric  dbl_ovrd=off  block_type=counter
  loop_stat : Outport
  loop_rdy : Outport  Port=2
  cap_loops : Outport  Port=3
  valid_loops : Outport  Port=4
  wires:
  time_counters/2(rdy) -> loop_rdy/1
  time_counters/1(stat) -> loop_stat/1
  valid_loop/1 -> valid_loops/1
  cap_loop/1 -> cap_loops/1
  timelim/1 -> time_counters/3(timelim)
  start/1 -> time_counters/2(start)
  cap_val/1 -> valid_loop/2
  cap_rdy/1 -> cap_loop/2
  rst/1 -> valid_loop/1, cap_loop/1, time_counters/1(rst)
  sigval/1 -> time_counters/4(sigval)
  force_stop/1 -> time_counters/5(force_stop)

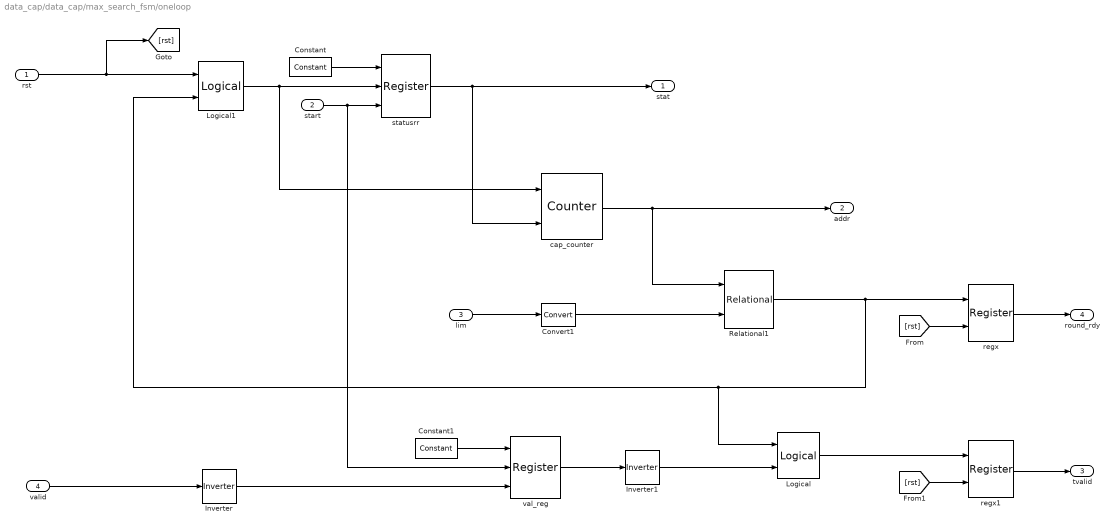
== system data_cap/data_cap/max_search_fsm/oneloop ==
  rst : Inport
  start : Inport  Port=2
  lim : Inport  Port=3
  valid : Inport  Port=4
  Constant : xbsIndex_r4/Constant  const=1  gui_display_data_type=Boolean  arith_type=Boolean  n_bits=1  bin_pt=0  preci_type=Single  exp_width=8  frac_width=24  explicit_period=off  period=1  equ=P=C  opselect=C  inp2=PCIN>>17  opr=+  inp1=P  carry=CIN  dbl_ovrd=off  block_type=constant
  Constant1 : xbsIndex_r4/Constant  const=1  gui_display_data_type=Boolean  arith_type=Boolean  n_bits=1  bin_pt=0  preci_type=Single  exp_width=8  frac_width=24  explicit_period=off  period=1  equ=P=C  opselect=C  inp2=PCIN>>17  opr=+  inp1=P  carry=CIN  dbl_ovrd=off  block_type=constant
  Convert1 : xbsIndex_r4/Convert  gui_display_data_type=Fixed-point  arith_type=Unsigned  n_bits=18  bin_pt=0  float_type=Single  exp_bits=8  fraction_bits=24  quantization=Truncate  overflow=Wrap  en=off  latency=0  pipeline=off  dbl_ovrd=off  block_type=convert
  Inverter : xbsIndex_r4/Inverter  en=off  latency=0  dbl_ovrd=off  block_type=inv
  Inverter1 : xbsIndex_r4/Inverter  en=off  latency=0  dbl_ovrd=off  block_type=inv
  Logical : xbsIndex_r4/Logical  logical_function=AND  inputs=2  en=off  latency=0  precision=Full  arith_type=Unsigned  n_bits=16  bin_pt=0  align_bp=on  dbl_ovrd=off  block_type=logical
  Logical1 : xbsIndex_r4/Logical  logical_function=OR  inputs=2  en=off  latency=0  precision=Full  arith_type=Unsigned  n_bits=16  bin_pt=0  align_bp=on  dbl_ovrd=off  block_type=logical
  Relational1 : xbsIndex_r4/Relational  mode=a=b  op_type=Bool  en=off  latency=0  dbl_ovrd=off  block_type=relational
  cap_counter : xbsIndex_r4/Counter  cnt_type=Free Running  cnt_to=Inf  operation=Up  start_count=0  cnt_by_val=1  arith_type=Unsigned  n_bits=18  bin_pt=0  load_pin=off  rst=on  en=on  explicit_period=on  period=1  use_behavioral_HDL=off  implementation=Fabric  dbl_ovrd=off  block_type=counter
  regx : xbsIndex_r4/Register  init=0  rst=on  en=off  dbl_ovrd=off  block_type=register
  regx1 : xbsIndex_r4/Register  init=0  rst=on  en=off  dbl_ovrd=off  block_type=register
  statusrr : xbsIndex_r4/Register  init=0  rst=on  en=on  dbl_ovrd=off  block_type=register
  val_reg : xbsIndex_r4/Register  init=0  rst=on  en=on  dbl_ovrd=off  block_type=register
  stat : Outport
  addr : Outport  Port=2
  tvalid : Outport  Port=3
  round_rdy : Outport  Port=4
  wires:
  [rst] -> regx1/2
  Logical/1 -> regx1/1
  [rst] -> regx/2
  regx/1 -> round_rdy/1
  val_reg/1 -> Inverter1/1
  Inverter/1 -> val_reg/3
  Constant1/1 -> val_reg/1
  start/1 -> val_reg/2, statusrr/3
  Constant/1 -> statusrr/1
  Logical1/1 -> statusrr/2, cap_counter/1
  rst/1 -> Logical1/1, [rst]
  Convert1/1 -> Relational1/2
  lim/1 -> Convert1/1
  Relational1/1 -> Logical1/2, Logical/1, regx/1
  valid/1 -> Inverter/1
  cap_counter/1 -> Relational1/1, addr/1
  statusrr/1 -> cap_counter/2, stat/1
  regx1/1 -> tvalid/1
  Inverter1/1 -> Logical/2

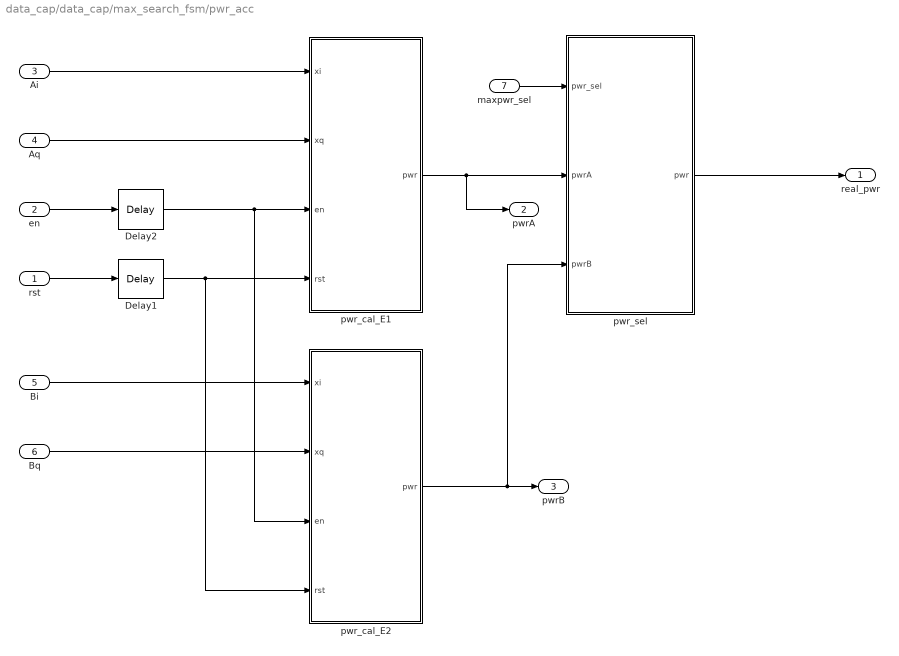
== system data_cap/data_cap/max_search_fsm/pwr_acc ==
  rst : Inport
  en : Inport  Port=2
  Ai : Inport  Port=3
  Aq : Inport  Port=4
  Bi : Inport  Port=5
  Bq : Inport  Port=6
  maxpwr_sel : Inport  Port=7
  Delay1 : xbsIndex_r4/Delay  rst=off  infoeditControl=Selection of Reset will increase slice count due to use of real FFs and instead of SRLs  en=off  latency=1  reg_retiming=off  dbl_ovrd=off  block_type=delay
  Delay2 : xbsIndex_r4/Delay  rst=off  infoeditControl=Selection of Reset will increase slice count due to use of real FFs and instead of SRLs  en=off  latency=1  reg_retiming=off  dbl_ovrd=off  block_type=delay
  pwr_cal_E1 : Subsystem
  pwr_cal_E2 : Subsystem
  pwr_sel : Subsystem
  real_pwr : Outport
  pwrA : Outport  Port=2
  pwrB : Outport  Port=3
  wires:
  en/1 -> Delay2/1
  rst/1 -> Delay1/1
  pwr_sel/1(pwr) -> real_pwr/1
  Ai/1 -> pwr_cal_E1/1(xi)
  Delay2/1 -> pwr_cal_E2/3(en), pwr_cal_E1/3(en)
  Delay1/1 -> pwr_cal_E2/4(rst), pwr_cal_E1/4(rst)
  Aq/1 -> pwr_cal_E1/2(xq)
  Bi/1 -> pwr_cal_E2/1(xi)
  Bq/1 -> pwr_cal_E2/2(xq)
  pwr_cal_E1/1(pwr) -> pwrA/1, pwr_sel/2(pwrA)
  pwr_cal_E2/1(pwr) -> pwrB/1, pwr_sel/3(pwrB)
  maxpwr_sel/1 -> pwr_sel/1(pwr_sel)

== system data_cap/data_cap/max_search_fsm/ram_control ==
  rst : Inport
  pwr_new : Inport  Port=2
  valid_trig : Inport  Port=3
  Logical : xbsIndex_r4/Logical  logical_function=AND  inputs=2  en=off  latency=0  precision=Full  arith_type=Unsigned  n_bits=16  bin_pt=0  align_bp=on  dbl_ovrd=off  block_type=logical
  Relational : xbsIndex_r4/Relational  mode=a>b  op_type=Bool  en=off  latency=0  dbl_ovrd=off  block_type=relational
  ram_switch : Subsystem
  regpwr : xbsIndex_r4/Register  init=0  rst=on  en=on  dbl_ovrd=off  block_type=register
  regx : xbsIndex_r4/Register  init=0  rst=on  en=off  dbl_ovrd=off  block_type=register
  ram_ind : Outport
  bigger_ind : Outport  Port=2
  wires:
  [rst] -> regx/2
  regx/1 -> bigger_ind/1
  valid_trig/1 -> Logical/2
  Relational/1 -> Logical/1
  pwr_new/1 -> Relational/1, regpwr/1
  regpwr/1 -> Relational/2
  rst/1 -> regpwr/2, ram_switch/1(rst), [rst]
  ram_switch/1(q) -> ram_ind/1
  Logical/1 -> regx/1, regpwr/3, ram_switch/2(tog)

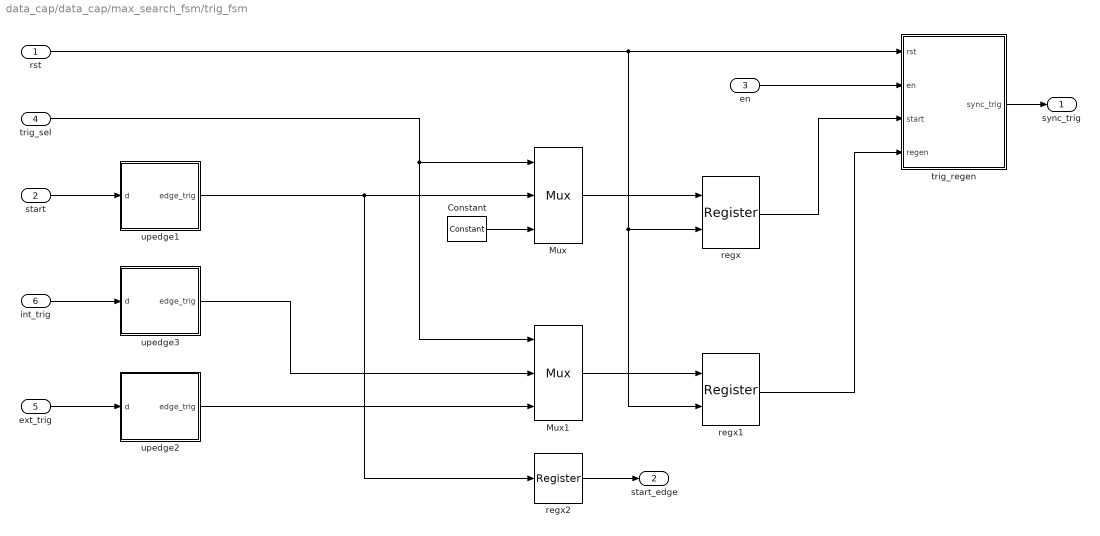
== system data_cap/data_cap/max_search_fsm/trig_fsm ==
  rst : Inport
  start : Inport  Port=2
  en : Inport  Port=3
  trig_sel : Inport  Port=4
  ext_trig : Inport  Port=5
  int_trig : Inport  Port=6
  Constant : xbsIndex_r4/Constant  const=0  gui_display_data_type=Boolean  arith_type=Boolean  n_bits=1  bin_pt=0  preci_type=Single  exp_width=8  frac_width=24  explicit_period=off  period=1  equ=P=C  opselect=C  inp2=PCIN>>17  opr=+  inp1=P  carry=CIN  dbl_ovrd=off  block_type=constant
  Mux : xbsIndex_r4/Mux  inputs=2  en=off  latency=0  precision=Full  arith_type=Unsigned  n_bits=16  bin_pt=14  quantization=Truncate  overflow=Wrap  dbl_ovrd=off  block_type=mux
  Mux1 : xbsIndex_r4/Mux  inputs=2  en=off  latency=0  precision=Full  arith_type=Unsigned  n_bits=16  bin_pt=14  quantization=Truncate  overflow=Wrap  dbl_ovrd=off  block_type=mux
  regx : xbsIndex_r4/Register  init=0  rst=on  en=off  dbl_ovrd=off  block_type=register
  regx1 : xbsIndex_r4/Register  init=0  rst=on  en=off  dbl_ovrd=off  block_type=register
  regx2 : xbsIndex_r4/Register  init=0  rst=off  en=off  dbl_ovrd=off  block_type=register
  trig_regen : Subsystem
  upedge1 : Subsystem
  upedge2 : Subsystem
  upedge3 : Subsystem
  sync_trig : Outport
  start_edge : Outport  Port=2
  wires:
  regx2/1 -> start_edge/1
  en/1 -> trig_regen/2(en)
  regx1/1 -> trig_regen/4(regen)
  regx/1 -> trig_regen/3(start)
  Mux1/1 -> regx1/1
  int_trig/1 -> upedge3/1(d)
  upedge2/1(edge_trig) -> Mux1/3
  Mux/1 -> regx/1
  upedge1/1(edge_trig) -> Mux/2, regx2/1
  trig_sel/1 -> Mux1/1, Mux/1
  Constant/1 -> Mux/3
  rst/1 -> trig_regen/1(rst), regx1/2, regx/2
  ext_trig/1 -> upedge2/1(d)
  start/1 -> upedge1/1(d)
  trig_regen/1(sync_trig) -> sync_trig/1
  upedge3/1(edge_trig) -> Mux1/2

== system data_cap/data_cap/ram_store/addr_conv ==
  d : Inport
  Concat : xbsIndex_r4/Concat  num_inputs=2  dbl_ovrd=off  block_type=concat
  Slice1 : xbsIndex_r4/Slice  nbits=1  boolean_output=off  mode=Upper Bit Location + Width  bit1=0  base1=MSB of Input  bit0=1  base0=LSB of Input  dbl_ovrd=off  block_type=slice
  Slice3 : xbsIndex_r4/Slice  nbits=cap_addr_width  boolean_output=off  mode=Lower Bit Location + Width  bit1=0  base1=MSB of Input  bit0=0  base0=LSB of Input  dbl_ovrd=off  block_type=slice
  q : Outport
  wires:
  Slice3/1 -> Concat/2
  d/1 -> Slice1/1, Slice3/1
  Slice1/1 -> Concat/1
  Concat/1 -> q/1

== system data_cap/data_cap/ram_store/addr_conv5 ==
  d : Inport
  Concat : xbsIndex_r4/Concat  num_inputs=2  dbl_ovrd=off  block_type=concat
  Slice1 : xbsIndex_r4/Slice  nbits=1  boolean_output=off  mode=Upper Bit Location + Width  bit1=0  base1=MSB of Input  bit0=1  base0=LSB of Input  dbl_ovrd=off  block_type=slice
  Slice3 : xbsIndex_r4/Slice  nbits=cap_addr_width  boolean_output=off  mode=Lower Bit Location + Width  bit1=0  base1=MSB of Input  bit0=0  base0=LSB of Input  dbl_ovrd=off  block_type=slice
  q : Outport
  wires:
  Slice3/1 -> Concat/2
  d/1 -> Slice1/1, Slice3/1
  Slice1/1 -> Concat/1
  Concat/1 -> q/1

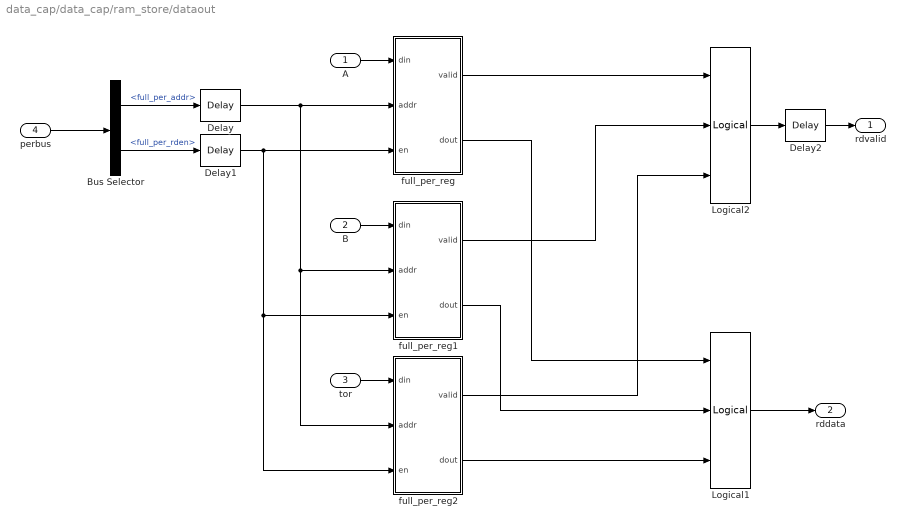
== system data_cap/data_cap/ram_store/dataout ==
  A : Inport
  B : Inport  Port=2
  tor : Inport  Port=3
  perbus : Inport  Port=4
  Bus Selector : BusSelector  OutputSignals=full_per_addr,full_per_rden
  Delay : xbsIndex_r4/Delay  rst=off  infoeditControl=Selection of Reset will increase slice count due to use of real FFs and instead of SRLs  en=off  latency=11  reg_retiming=off  dbl_ovrd=off  block_type=delay
  Delay1 : xbsIndex_r4/Delay  rst=off  infoeditControl=Selection of Reset will increase slice count due to use of real FFs and instead of SRLs  en=off  latency=11  reg_retiming=off  dbl_ovrd=off  block_type=delay
  Delay2 : xbsIndex_r4/Delay  rst=off  infoeditControl=Selection of Reset will increase slice count due to use of real FFs and instead of SRLs  en=off  latency=1  reg_retiming=off  dbl_ovrd=off  block_type=delay
  Logical1 : xbsIndex_r4/Logical  logical_function=OR  inputs=3  en=off  latency=1  precision=Full  arith_type=Unsigned  n_bits=16  bin_pt=0  align_bp=on  dbl_ovrd=off  block_type=logical
  Logical2 : xbsIndex_r4/Logical  logical_function=OR  inputs=3  en=off  latency=1  precision=Full  arith_type=Unsigned  n_bits=16  bin_pt=0  align_bp=on  dbl_ovrd=off  block_type=logical
  full_per_reg : Subsystem
  full_per_reg1 : Subsystem
  full_per_reg2 : Subsystem
  rdvalid : Outport
  rddata : Outport  Port=2
  wires:
  perbus/1 -> Bus Selector/1
  Bus Selector/1 -> Delay/1  "<full_per_addr>"
  Bus Selector/2 -> Delay1/1  "<full_per_rden>"
  A/1 -> full_per_reg/1(din)
  B/1 -> full_per_reg1/1(din)
  Logical2/1 -> Delay2/1
  full_per_reg/2(dout) -> Logical1/1
  full_per_reg/1(valid) -> Logical2/1
  full_per_reg1/1(valid) -> Logical2/2
  full_per_reg1/2(dout) -> Logical1/2
  tor/1 -> full_per_reg2/1(din)
  full_per_reg2/1(valid) -> Logical2/3
  full_per_reg2/2(dout) -> Logical1/3
  Logical1/1 -> rddata/1
  Delay/1 -> full_per_reg2/2(addr), full_per_reg1/2(addr), full_per_reg/2(addr)
  Delay1/1 -> full_per_reg2/3(en), full_per_reg1/3(en), full_per_reg/3(en)
  Delay2/1 -> rdvalid/1

== system data_cap/data_cap/ram_store/ram0_ctrl ==
  cap_ramsel : Inport
  cap_addr : Inport  Port=2
  cap_wren : Inport  Port=3
  per_addr : Inport  Port=4
  txi : Inport  Port=5
  txq : Inport  Port=6
  Concat1 : xbsIndex_r4/Concat  num_inputs=2  dbl_ovrd=off  block_type=concat
  Concat2 : xbsIndex_r4/Concat  num_inputs=2  dbl_ovrd=off  block_type=concat
  Inverter : xbsIndex_r4/Inverter  en=off  latency=1  dbl_ovrd=off  block_type=inv
  iqcomb_32b : Subsystem
  addr : Outport
  din : Outport  Port=2
  wren : Outport  Port=3
  rd_addr : Outport  Port=4
  wires:
  txq/1 -> iqcomb_32b/2(dq)
  txi/1 -> iqcomb_32b/1(di)
  cap_wren/1 -> wren/1
  Inverter/1 -> Concat2/1
  cap_addr/1 -> Concat1/2
  cap_ramsel/1 -> Inverter/1, Concat1/1
  per_addr/1 -> Concat2/2
  Concat1/1 -> addr/1
  Concat2/1 -> rd_addr/1
  iqcomb_32b/1(q) -> din/1

== system data_cap/data_cap/ram_store/ram0_ctrl1 ==
  cap_ramsel : Inport
  cap_addr : Inport  Port=2
  cap_wren : Inport  Port=3
  per_addr : Inport  Port=4
  txi : Inport  Port=5
  txq : Inport  Port=6
  Concat1 : xbsIndex_r4/Concat  num_inputs=2  dbl_ovrd=off  block_type=concat
  Concat2 : xbsIndex_r4/Concat  num_inputs=2  dbl_ovrd=off  block_type=concat
  Inverter : xbsIndex_r4/Inverter  en=off  latency=1  dbl_ovrd=off  block_type=inv
  iqcomb_32b : Subsystem
  addr : Outport
  din : Outport  Port=2
  wren : Outport  Port=3
  rd_addr : Outport  Port=4
  wires:
  Concat2/1 -> rd_addr/1
  per_addr/1 -> Concat2/2
  Inverter/1 -> Concat2/1
  cap_wren/1 -> wren/1
  txi/1 -> iqcomb_32b/1(di)
  txq/1 -> iqcomb_32b/2(dq)
  iqcomb_32b/1(q) -> din/1
  cap_ramsel/1 -> Concat1/1, Inverter/1
  cap_addr/1 -> Concat1/2
  Concat1/1 -> addr/1
